simulink model "test2"  (R2015a)
settings: Solver=ode3  StartTime=0.0  StopTime=10.0  RelTol=1e-3
libraries: PoliArd x5
settings Model: ExtModeTrigDuration=2  Creator=User  LastModifiedBy=dell
settings OptimizationCC: OptimizeModelRefInitCode=on  LifeSpan=1
settings DebuggingCC: UnderspecifiedInitializationDetection=Classic  MergeDetectMultiDrivingBlocksExec=none
settings HardwareCC: ProdLargestAtomicInteger=Long  ProdLargestAtomicFloat=Double  ProdEndianess=LittleEndian  ProdHWDeviceType=ARM Compatible->ARM Cortex
settings RTWCC: SystemTargetFile=realtime.tlc  GenerateMakefile=off  TemplateMakefile=realtime.tmf  Description=Run on Target Hardware  RTWVerbose=off
settings ERTTargetCC: CombineOutputUpdateFcns=off  ExtModeTransport=3  ExtModeMexFile=ext_serial_win32_comm_rtt  ExtModeMexArgs=0 1 9600  ERTSrcFileBannerTemplate=realtime_code_template.cgt  ERTHdrFileBannerTemplate=realtime_code_template.cgt  ERTDataSrcFileTemplate=realtime_code_template.cgt  ERTDataHdrFileTemplate=realtime_code_template.cgt  ERTCustomFileTemplate=realtime_file_process.tlc

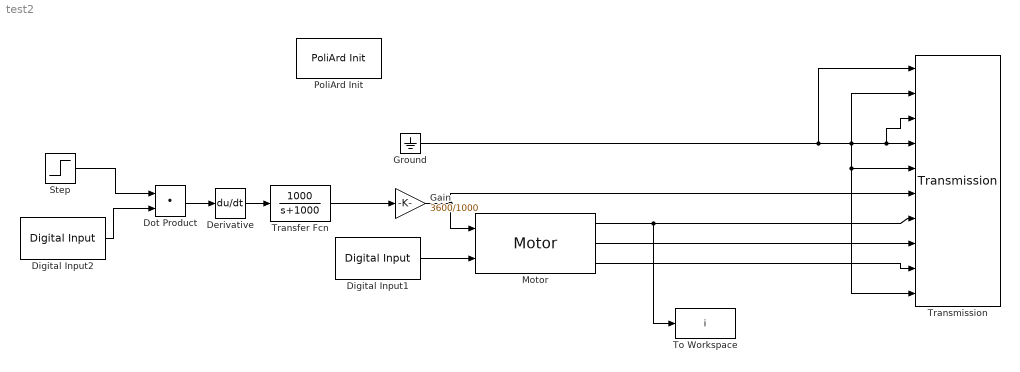
== system test2 ==
  Derivative : Derivative
  Digital Input1 : PoliArd/Digital Input  DI_pin=3  DIsample=-1
  Digital Input2 : PoliArd/Digital Input  DI_pin=2  DIsample=-1
  Dot Product : DotProduct  InputSameDT=on  OutDataTypeStr=Inherit: Inherit via internal rule
  Gain : Gain  Gain=3600/1000
  Ground : Ground
  Motor : PoliArd/Motor  MotorID=1  DC_bus_mask=12  dt_mot=-1
  PoliArd Init : PoliArd/PoliArd Init
  Step : Step  Time=0  SampleTime=0
  To Workspace : ToWorkspace  VariableName=i  SaveFormat=Timeseries  SampleTime=-1
  Transfer Fcn : TransferFcn  Numerator=[1000]  Denominator=[1 1000]
  Transmission : PoliArd/Transmission  sample_freq=100  sig_to_send=6
  wires:
  Digital Input1/1 -> Motor/2
  Ground/1 -> Transmission/1, Transmission/2, Transmission/10, Transmission/5, Transmission/3, Transmission/4
  Motor/1 -> To Workspace/1, Transmission/7
  Gain/1 -> Transmission/6, Motor/1
  Motor/3 -> Transmission/9
  Motor/2 -> Transmission/8
  Transfer Fcn/1 -> Gain/1
  Step/1 -> Dot Product/1
  Digital Input2/1 -> Dot Product/2
  Derivative/1 -> Transfer Fcn/1
  Dot Product/1 -> Derivative/1
